simulink model "pamSimu"  (R2016a)
settings: Solver=VariableStepAuto  StartTime=0.0  StopTime=10.0  RelTol=1e-3
libraries: commdigbbndam3 x1
settings Model: Creator=ahpar  LastModifiedBy=ahpar

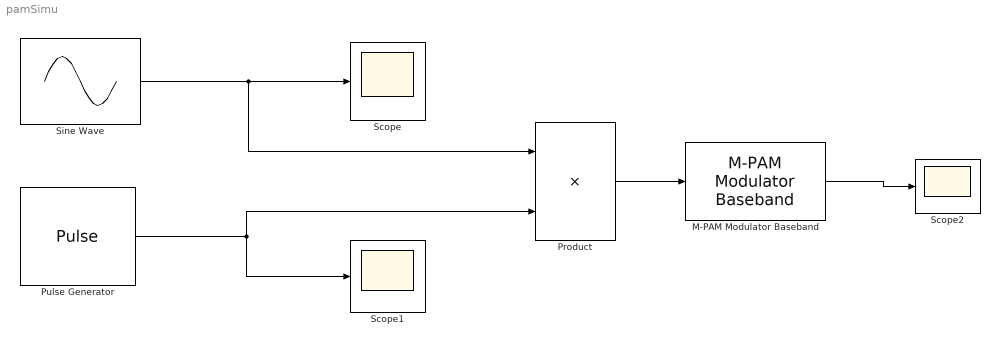
== system pamSimu ==
  M-PAM Modulator Baseband : commdigbbndam3/M-PAM Modulator Baseband  M=2  InType=Integer  Enc=Gray  PowType=Average Power  MinDist=2  AvgPow=1  PeakPow=1  outDtype=double  outWordLen=16  outUDDataType=sfix(16)  outFracLenMode=Best precision  outFracLen=15  outDataTypeStr=double  outLastDataTypeStr=double
  Product : Product
  Pulse Generator : DiscretePulseGenerator  Period=10  PulseWidth=5
  Scope : Scope
  Scope1 : Scope
  Scope2 : Scope
  Sine Wave : Sin  SampleTime=0
  wires:
  Sine Wave/1 -> Product/1, Scope/1
  Pulse Generator/1 -> Scope1/1, Product/2
  Product/1 -> M-PAM Modulator Baseband/1
  M-PAM Modulator Baseband/1 -> Scope2/1
